simulink model "Final_Model_Building_2_AirflowAdded_BufferMode"  (R2022a)
settings: Solver=FixedStepAuto  StartTime=0.0  StopTime=24*3600  FixedStep=5  RelTol=1e-3
values from neighbouring files (symbols this model uses):
  Aux_Threshold = 52    [Setup_Code_EWASP_VC.m]
  buildingAge = 2005    [Setup_Code_EWASP_VC.m]
  ceilingHeight = 2.4    [Setup_Code_EWASP_VC.m]
  conductiveHconnectMatrix = [ ... (first row only)    [Setup_Code_EWASP_VC.m]
  cRoofGreen = 100000    [Setup_Code_EWASP_VC.m]
  Defrost_After_Time = 30    [Setup_Code_EWASP_VC.m]
  DHWDemandProfile = occFreegainHotwaterElecTestPassiveOcc3(:,3)    [Setup_Code_EWASP_VC.m]
  Elec_Max = Elec_Max*(30/24.2)    [Setup_Code_EWASP_VC.m]
  Elec_Mid = Elec_Mid*(30/24.2)    [Setup_Code_EWASP_VC.m]
  Elec_Min = Elec_Min*(30/24.2)    [Setup_Code_EWASP_VC.m]
  ElecDemandProfile = occFreegainHotwaterElecTestPassiveOcc3(:,4)    [Setup_Code_EWASP_VC.m]
  ElecFixed = [Elec_Max(6,2) Elec_Max(6,4) Elec_Max(6,6) Elec_Max(6,7) ... (first row only)    [Setup_Code_EWASP_VC.m]
  floorOrCeilingArea = floorOrCeilingArea*1.15    [Setup_Code_EWASP_VC.m]
  freegain = occFreegainHotwaterElecTestPassiveOcc3(:,2)-max(occupancy)*25    [Setup_Code_EWASP_VC.m]
  furnitureModelOn = 1    [Setup_Code_EWASP_VC.m]
  Heat_Max = Heat_Max*(30/24.2)    [Setup_Code_EWASP_VC.m]
  Heat_Mid = Heat_Mid*(30/24.2)    [Setup_Code_EWASP_VC.m]
  Heat_Min = Heat_Min*(30/24.2)    [Setup_Code_EWASP_VC.m]
  HeatFixed = [Heat_Max(6,2) Heat_Max(6,4) Heat_Max(6,6) Heat_Max(6,7) ... (first row only)    [Setup_Code_EWASP_VC.m]
  HeatingOnProfile = repmat(HeatingOnProfile,365,1)    [Setup_Code_EWASP_VC.m]
  HEX_ReturnLowerLimit = 52.5    [Setup_Code_EWASP_VC.m]
  HEX_ReturnUpperLimit = 55    [Setup_Code_EWASP_VC.m]
  LeakMultiplier = 1+(2*(rand()-0.5)/10)    [Setup_Code_EWASP_VC.m]
  maxOcc = max(occupancyProfile)    [Setup_Code_EWASP_VC.m]
  NESW_wallArea = max(NESW_Lengths*ceilingHeight-NESW_Windows,0)    [Setup_Code_EWASP_VC.m]
  NESW_Windows = [ ... (first row only)    [Setup_Code_EWASP_VC.m]
  numRooms = roomCount    [Setup_Code_EWASP_VC.m]
  occupancy = occupancyProfile    [Setup_Code_EWASP_VC.m]
  offsetDays = 0    [Setup_Code_EWASP_VC.m]
  overChargeSeries = repmat(overChargeSeries,365,1)    [Setup_Code_EWASP_VC.m]
  pumpChoice = pumpChoices(MinIndex,1)    [Setup_Code_EWASP_VC.m]
  pumpRamp = 180    [Setup_Code_EWASP_VC.m]
  RoofIrradiance = Flat_NS_EW_RoofIrradiance(:,1)    [Setup_Code_EWASP_VC.m]
  roofStartTemp = ones(11,1)*20    [Setup_Code_EWASP_VC.m]
  rooftype = 0    [Setup_Code_EWASP_VC.m]
  RoomDataMatrix = [zeros(1,12);ones(1,12)*wallDensity;zeros(1,12);ones(1,12)*wallU;ones(1,12)*windowU;ones(1,12)*floorU;ones(1,12)*ceilingU;zeros(1,12);windowArea, 0;floorOrCeilingArea;zeros(1,12);floorOrCeilingArea*ceilingHeight]    [Setup_Code_EWASP_VC.m]
  roomVol = roomVol*1.15    [Setup_Code_EWASP_VC.m]
  slabStartTemp = (GroundTempTimeSeries(offsetDays*1440+1,1)+thermostatSetting)/2    [Setup_Code_EWASP_VC.m]
  SlackRequest = zeros(1440,1)    [Setup_Code_EWASP_VC.m]
  SolarThermalExists = 0    [Setup_Code_EWASP_VC.m]
  SourceFixed = HeatFixed-ElecFixed    [Setup_Code_EWASP_VC.m]
  StateSeries = StateSeriesGenerator(22,7,1)    [Setup_Code_EWASP_VC.m]
  Tank_Lower_Temp = 49.5    [Setup_Code_EWASP_VC.m]
  Tank_Upper_Temp = 52    [Setup_Code_EWASP_VC.m]
  Tank_Volume_m3 = 0.15    [Setup_Code_EWASP_VC.m]
  TankHeatHour = randi([1 5])-1    [Setup_Code_EWASP_VC.m]
  upDown = [0;0;0;0;1;1;1;1;1;1;1]    [Setup_Code_EWASP_VC.m]
  wallStartTempExt = thermostatSetting*(0.266+0.00215*outdoorStartTemp+0.018*wallU+0.00113*outdoorStartTemp*wallU+0.0068*wallU^2)    [Setup_Code_EWASP_VC.m]
undefined symbols (not defined in the file or in its folder): a, ceilingU, condUDMatrix, convUDMatrix, deltaPEXPANDED_E, deltaPEXPANDED_E2, deltaPEXPANDED_N, deltaPEXPANDED_N2, deltaPEXPANDED_S, deltaPEXPANDED_S2, deltaPEXPANDED_W, deltaPEXPANDED_W2, DesiredDHWTemp, DesiredFlowTempVsInOutDeltaTemp, DiffuseHorizontal, DiscIntNeverNeededParam, DNI, dwnAndConcrete, ExtractRates, GroundTempTimeSeries, HCM, HCM2, HCM_closed, HCM_closed2, intermediateU, IsTop, massFlowMatrix, mechEfficiency, neighbourMatrix, numericalRoomUse, RadiatorMatrix, room2roomflowmatrix_E, room2roomflowmatrix_E2, room2roomflowmatrix_N, room2roomflowmatrix_N2, room2roomflowmatrix_S, room2roomflowmatrix_S2, room2roomflowmatrix_W, room2roomflowmatrix_W2, StateAirInEXPANDED_E, StateAirInEXPANDED_E2, StateAirInEXPANDED_N, StateAirInEXPANDED_N2, StateAirInEXPANDED_S, StateAirInEXPANDED_S2, StateAirInEXPANDED_W, StateAirInEXPANDED_W2, StateAirOutEXPANDED_E, StateAirOutEXPANDED_E2, StateAirOutEXPANDED_N, StateAirOutEXPANDED_N2, StateAirOutEXPANDED_S, StateAirOutEXPANDED_S2, StateAirOutEXPANDED_W, StateAirOutEXPANDED_W2, tankExists, TemperatureSeries, ThermostatBand, ThermostatSetting, Tin1 ... (+10)
libraries: simulink x6, dspsigops x4, dspmtrx3 x4, powerlib_meascontrol x3, carnot x3, dspstat3 x2
(part 7 of 29)

== system Final_Model_Building_2_AirflowAdded_BufferMode/GSHP_Subsystem/Subsystem3 ==
  note: only required to allow me to send the
      | same signal to 2 different outputs
  note: SH GSHP
  In1 : Inport
  In2 : Inport  Port=2
  In3 : Inport  Port=3
  In4 : Inport  Port=4
  In5 : Inport  Port=5
  In6 : Inport  Port=6
  In7 : Inport  Port=7
  Bus Selector1 : BusSelector  OutputSignals=Pelec  OutputAsBus=on
  Clock4 : Clock
  Data Type Conversion2 : DataTypeConversion  OutDataTypeStr=double  SaturateOnIntegerOverflow=off  RndMeth=Floor
  Data Type Conversion3 : DataTypeConversion  OutDataTypeStr=double  SaturateOnIntegerOverflow=off  RndMeth=Floor
  Data Type Conversion4 : DataTypeConversion  OutDataTypeStr=double  SaturateOnIntegerOverflow=off  RndMeth=Floor
  Ground_Source_Heat_Exchanger1 : Subsystem  AncestorBlock=carnot/Source/Heat_Pump/Ground_Source_Heat_Exchanger  mask(vertical ground source heat exchanger){Jahresmitteltemp_C=12, TGrad=0.025, lambdaErde=5, cpErde=11000, rhoErde=2500, lambdaFill=5, cpFill=1000, rhoFill=2000, Sondelaenge=100, B=10, Sondendurchmesser=0.032, Bohrdurchmesser=0.18, sondenfall=2 probes B/H = 0.1, np=2, DimAxi=10, DimRad=10, Gitterfaktor=2.5}
      mask prompts: Jahresmitteltemp_C "Average annual outdoor temperature  in °C"; TGrad "Temperature gradient in K/m, typical 0.025..0.04"; lambdaErde "Thermal conductivity ground in W/m/K"; cpErde "Heat capacity of the ground in J/kg/K"; rhoErde "Denstiy of the ground in kg/m³"; lambdaFill "Thermal conductivity filling in W/m/K"; cpFill "Heat capacity of the filling in J/kg/K"; rhoFill "Denstiy of the filling in kg/m³"; Sondelaenge "H: Length of earth probe in m"; B "B: probe distance in m"; Sondendurchmesser "Diameter of tube in m"; Bohrdurchmesser "Diameter of drilled hole in m"; sondenfall "Field geometry"; np "Number of parallel tubes"; DimAxi "No. of nodes in axial direction (typical 10)"; DimRad "No. of nodes in radial direction (typical 10)"; Gitterfaktor "grid factor (typical 2.5)"
      mask help:
      | The CARNOT EWS model is a transient model for dynamic simulation of borehole heat exchangers or so-called vertical ground heat exchangers. The model is based on the equations described by [Huber97] and has been implemented using the state space model of Matlab/Simulink [Bianchi06].
      | Bianchi M. A., Adaptive modellbasierte prädiktive Regelung einer Kleinwärmepumenanlage Diss. ETH Zuerich, No. 16892, 2006
      | Huber A, Schuler O., Berechnungsmodul für Erdwärmesonden (EWS). ENET Bericht Nr. 9658807-1, 1997
      mask init:
      | % Sets the parameters for the model
      | % ***********************************************************************
      | % This file is part of the CARNOT Blockset.
      | %   CARNOT is free software: you can redistribute it and/or modify
      | %   it under the terms of the GNU Lesser General Public License as published by
      | %   the Free Software Foundation, either version 3 of the License, or
      | %   (at your option) any later version.
      | %   CARNOT is distributed in the hope that it will be useful,
      | %   but WITHOUT ANY WARRANTY; without even the implied warranty of
      | %   MERCHANTABILITY or FITNESS FOR A PARTICULAR PURPOSE.  See the
      | %   GNU Lesser General Public License for more details.
      | %   You should have received a copy (copying_lesser.txt) of the 
      | %   GNU Lesser General Public License along with CARNOT.  
      | %   If not, see <http://www.gnu.org/licenses/>.
      | %  
      | % **********************************************************************
      | % author list:      fab -> Fabian Ochs
      | %                   hf  -> Bernd Hafner
      | %
      | % version: CarnotVersion.MajorVersionOfFunction.SubversionOfFunction
      | %
      | % Version  Author  Changes                                     Date
      | % 5.1.0    fab     created, based on Diss. Bianchi ETH Zurich  01dec2012
      | % 5.1.1    hf      adapted to carnot input and output struct.  04mar2013 
      | %
      | % Copyright (c) 2012 TU Insbruck, Fabian Ochs
      | 
      | startfall = 2; % 2: g-function
      | mdot = 0.5;
      | teta_in = 1;
      | Massenstrom = mdot/np;
      | Qdot0 = 5000;
      | t_start = 50*8560*3600;
      | 
      | % Geometry
      | Dicke_Sondenrohr = 0.003;
      | lambda_Sondenrohr = 0.48;
      | Bu = .1293;
      | 
      | % Ground Properties
      | aErde = lambdaErde/(rhoErde*cpErde);
      | 
      | % Fluid
      | teta_m = 2; 
      | p0 = 1E5;
      | fluid = 5;
      | mix = 0.25;
      | 
      | Jahresmitteltemp=Jahresmitteltemp_C + 273.15;
      | Bodenerwaermung=1;                          % 0°C
      | Bodentemp=Jahresmitteltemp+Bodenerwaermung; % K
      | 
      | % Calculation
      | lambdaSole=thermal_conductivity(teta_m,p0,fluid,mix);%W/(m K)
      | cpSole=heat_capacity(teta_m,p0,fluid,mix);                                % J/Kg*K
      | rhoSole=density(teta_m,p0,fluid,mix);%kg/m^3
      | vSole=kinematic_viscosity(teta_m,p0,fluid,mix);                             % m2/s
      | 
      | Pr=vSole*rhoSole*cpSole/lambdaSole;
      | rb = Bohrdurchmesser/2;
      | rm = B/2;
      | Rechenradius = rm;
      | Dl=Sondelaenge/DimAxi*2;    
      | 
      | rs=Sondendurchmesser/2;
      | r0 = rs-Dicke_Sondenrohr; % Innenradius
      | r1=Bohrdurchmesser/2;
      | r2=r1+(Rechenradius-r1)*(1-Gitterfaktor)/(1-Gitterfaktor^(DimRad-1))*Gitterfaktor^0;
      | 
      | rz1=((r1^2+r0^2)/2)^0.5;
      | rz2=((r2^2+r1^2)/2)^0.5;
      | 
      | mcpSole=2*cpSole*rhoSole*pi*Dl*(Sondendurchmesser/2)^2;
      | Di = Sondendurchmesser - 2 * Dicke_Sondenrohr;
      | Geschw_Sole= Massenstrom/rhoSole/(Di/2)^2/pi/2; % 2: double U
      | 
      | Vdot = Massenstrom/rhoSole;
      | A_p = (Di/2)^2/pi/2;
      | 
      | Re=Geschw_Sole*Di/vSole;
      | Druckverlust= 1/(1.82*log10(Re)-1.64)^2;
      | K1=1+27.2*Druckverlust/8;
      | K1_o=1.106886;
      | K2=11.7+1.8*Pr^(-1.3);
      | Druckverlust_o=0.031437;
      | St_o= Druckverlust_o/8/(K1_o+K2*(Druckverlust_o/8)^0.5*(Pr^(2/3)-1));
      | Nu_o=St_o*10000*Pr;
      | St= Druckverlust/8/(K1+K2*(Druckverlust/8)^0.5*(Pr^(2/3)-1));
      | 
      | % acc. Hellström    
      | b = Bu/(2*r1);
      | b_max = 1-rs/r1;
      | b_min = rs/r1;
      | sigma = (lambdaFill-lambdaErde)/(lambdaErde+lambdaFill);
      | A = pi*r0^2;
      | vs = Massenstrom/2/rhoSole/A;
      | zeta = 1/((1.82*log10(Re)-1.64)^2);
      | K1 = 1+27.2*zeta/8;
      | K2 = 11.7+1.8*Pr^(-1/3); 
      | R_s = 1/(2*pi*lambda_Sondenrohr)*log(rs/r0);
      |     
      | Nu_turbulent=St*Re*Pr;        
      | Nu_laminar=4.36;
      | 
      | if Re>=10000,
      |     Nu =(zeta/8)*Re*Pr/(K1+K2*(zeta/8)^.5*(Pr^(2/3)-1));
      | elseif Re<10000 && Re>2300
      |     Nu = Nu_laminar*exp(log(Nu_o/Nu_laminar)*log(Re/2300)/log(10000/2300));
      | elseif Re<=2300,
      |     Nu=Nu_laminar;        
      | end
      |     
      | alpha = Nu*lambdaSole/(2*r0);
      | alpha_eff = (1/alpha+r0/lambda_Sondenrohr*log(rs/r0))^-1;
      | alpha0 = lambdaSole/(Di/2*(1-0.5^0.5));
      | alpha0_eff = (1/alpha0+r0/lambda_Sondenrohr*log(rs/r0))^-1;
      | 
      | R_a = 1/(8*pi*alpha*r0);
      | beta = lambdaFill*(1/(r0*alpha)+1/lambda_Sondenrohr*log(rs/r0));
      | 
      | R1_EWS=0.25*(1/(2*pi*alpha_eff*r0*Dl)+1/(2*pi*lambdaFill*Dl)*log((r1-rz1)/r0));
      | R2_EWS=1/(2*pi*Dl)*(1/lambdaFill*log(r1/rz1)+1/lambdaErde*log(rz2/r1));        
      | R10_EWS=0.25*(1/(2*pi*alpha0_eff*r0*Dl)+1/(2*pi*lambdaFill*Dl)*log((r1-rz1)/r0));
      | R20_EWS=1/(2*pi*Dl)*(1/lambdaFill*log(r1/rz1)+1/lambdaErde*log(rz2/r1));        
      | 
      | Ra = 1/(pi*lambdaFill)*(log((2^.5*b*r1)/r0)-1/2*log((2*b*r1)/r0)-1/2*sigma*log((1-b^4)/(1+b^4)))+(1/(2*pi*r0*alpha))+R_s;
      | Rb = (1/(8*pi*lambdaFill))*(beta+log(r1/r0)+log(r1/Bu)+sigma*log(r1^4/(r1^4-Bu^4/16))-(r0^2/Bu^2*(1-sigma*(Bu^474)/(r1^4-Bu^4/16)^2))/((1+beta)/(1-beta)+r0^2/Bu^2*(1+sigma*Bu^4*r1^4/(r1^4-Bu^4/16)^2)));
      | Ra0 = 1/(pi*lambdaFill)*(log((2^.5*b*r1)/r0)-1/2*log((2*b*r1)/r0)-1/2*sigma*log((1-b^4)/(1+b^4)))+(1/(2*pi*r0*alpha0))+R_s;
      | Rb0 = (1/(8*pi*lambdaFill))*(beta+log(r1/r0)+log(r1/Bu)+sigma*log(r1^4/(r1^4-Bu^4/16))-(r0^2/Bu^2*(1-sigma*(Bu^474)/(r1^4-Bu^4/16)^2))/((1+beta)/(1-beta)+r0^2/Bu^2*(1+sigma*Bu^4*r1^4/(r1^4-Bu^4/16)^2)));
      | 
      | if Ra < 4 * Rb
      |     R1 = Ra/(4*Dl);
      |     R2 = (Rb-Ra/4)/Dl+(2*pi*Dl*lambdaErde)^-1*log(rz2/r1);
      |     R10 = Ra0/(4*Dl);
      |     R20 = (Rb0-Ra0/4)/Dl+(2*pi*Dl*lambdaErde)^-1*log(rz2/r1);        
      | else
      |     R1 = R1_EWS;
      |     R2 = R2_EWS;
      |     R10 = R10_EWS;
      |     R20 = R20_EWS;
      | end
      |     
      | % temperaturverlauf axialer richtung
      | L0=cpSole*Massenstrom;      % konstant
      | L00 = 0.0;
      | L1=1/R1;
      | L2=1/R2;
      | L10=1/R10;
      | L20=1/R20;
      | 
      | % matrizen Ad,Bd,Cd,Dd für Tdown
      | Ad=zeros(DimAxi/2,DimAxi/2);
      | Ad0=zeros(DimAxi/2,DimAxi/2);
      | for h=1:DimAxi/2,
      |     Ad(h,h)=-(L0/(mcpSole)+L1/(2*mcpSole));
      |     Ad0(h,h)=-(L00/(mcpSole)+L10/(2*mcpSole));
      | end
      |   
      | for h=1:DimAxi/2-1,
      |     Ad(h+1,h)=L0/(mcpSole);
      |     Ad0(h+1,h)=L00/(mcpSole);
      | end
      | 
      | Bd=zeros(DimAxi/2,DimAxi/2+1);
      | Bd0=zeros(DimAxi/2,DimAxi/2+1);
      | Bd(1,1)=L0/(mcpSole);
      | Bd0(1,1)=L00/(mcpSole);
      | 
      | for h=1:DimAxi/2,
      |     Bd(h,h+1)=L1/(2*mcpSole);
      |     Bd0(h,h+1)=L10/(2*mcpSole);
      | end
      | 
      | Cd=eye(DimAxi/2);
      | Dd=zeros(DimAxi/2,DimAxi/2+1);
      | 
      | % matrizen Au,Bu,Cu,Du für Tup
      | Au=zeros(DimAxi/2,DimAxi/2);
      | Au0=zeros(DimAxi/2,DimAxi/2);
      | for h=1:DimAxi/2,
      |     Au(h,h)=-(L0/(mcpSole)+L1/(2*mcpSole));
      |     Au0(h,h)=-(L00/(mcpSole)+L10/(2*mcpSole));
      | end
      |   
      | for h=1:DimAxi/2-1,
      |     Au(h+1,h)=L0/(mcpSole);
      |     Au0(h+1,h)=L00/(mcpSole);
      | end
      | 
      | Bu=zeros(DimAxi/2,DimAxi/2+1);
      | Bu0=zeros(DimAxi/2,DimAxi/2+1);
      | Bu(1,1)=L0/(mcpSole);
      | Bu0(1,1)=L00/(mcpSole);
      | for h=1:DimAxi/2,
      |     Bu(h,h+1)=L1/(2*mcpSole);
      |     Bu0(h,h+1)=L10/(2*mcpSole);
      | end
      | 
      | Cu=Cd;
      | Du=zeros(DimAxi/2,DimAxi/2+1);
      | 
      | % berechnung von Tradial, von Luzi Valär
      | Dim1=(DimRad-2)*DimAxi/2;
      | r = zeros(1:DimRad);
      | r(1)=Bohrdurchmesser/2;
      | r(2)=r2;
      | for h =3:DimRad,
      |     r(h)=r(h-1)+(Rechenradius-r1)*(1-Gitterfaktor)/(1-Gitterfaktor^(DimRad-1))*Gitterfaktor^(h-2);
      | end
      |     
      | rz = zeros(1:DimRad);
      | rz(1)=((r(1)^2+r0^2)/2)^0.5;
      | for h = 2:DimRad,
      |     rz(h)=((r(h)^2+r(h-1)^2)/2)^0.5;
      | end
      | 
      | L = zeros(1:DimRad);
      | L(1)=L1; 
      | L(2)=L2;
      | for h = 3:DimRad-1,
      |     L(h)=1/(1/(2*pi*Dl)*(1/lambdaErde*log(rz(h)/rz(h-1))));
      | end
      | L(DimRad)=1/(1/(2*pi*Dl)*(1/lambdaErde*log(r(DimRad)/rz(DimRad-1))));
      | 
      | 
      | C = zeros(1:DimRad);
      | C(1)=cpFill*rhoFill*pi*(r(1)^2-4*r0^2)*Dl;
      | for h = 2:DimRad,
      |     C(h)=cpErde*rhoErde*pi*(r(h)^2-r(h-1)^2)*Dl;
      | end
      | 
      | 
      | a=zeros(DimRad-2,DimRad-2);
      | for h = 1:DimRad-2,
      |     a(h,h)=(-L(h)-L(h+1))/C(h);
      | end
      | for h = 1:DimRad-3,
      |     a(h,h+1)=L(h+1)/C(h);
      |     a(h+1,h)=L(h+1)/C(h+1);
      | end
      | 
      | b=zeros(DimRad-2,2);
      |     b(1,1)=L(1)/C(1);
      |     b(DimRad-2,2)=L(DimRad-1)/C(DimRad-2);
      |     
      | %%%%%%%%%%%%%%%%%%%%%%%%%%%%%%%%%%%%%%%%%%%%%%%%%%% 
      |     
      | Ar=a;
      | Ar(DimRad-1:2*(DimRad-2),DimRad-1:2*(DimRad-2))=a;
      |     
      | for h=2:DimAxi/2-1,
      |     Ar(h*(DimRad-2)+1:(h+1)*(DimRad-2),h*(DimRad-2)+1:(h+1)*(DimRad-2))=a;
      | 
      | end  
      | 
      | Br=b;
      | 
      | for h=1:DimAxi/2-1,
      |     Br(h*(DimRad-2)+1:(h+1)*(DimRad-2),2*h+1:2*h+2)=b;   
      | end
      |     
      | 
      | Cr=eye((DimRad-2)*DimAxi/2);
      | Dr=zeros((DimRad-2)*DimAxi/2,DimAxi);
      | 
      | % andere matrizen
      | Cdl=zeros(DimAxi/2,1);
      | Cdl(DimAxi/2,1)=1;
      | Cdl=Cdl';
      | 
      | c1=zeros(DimAxi/2,Dim1);
      | for h=1:DimAxi/2,
      |     c1(1,1)=1;
      |     c1(h,(h-1)*(DimRad-2)+1)=1;
      | end
      | 
      | c31=zeros(1,DimAxi/2);
      | c3(1,1)=1;
      | for h=1:DimAxi/2-1,
      |     c3(1+2*h,1+h)=1;
      | end
      | 
      | c33=zeros(DimAxi,DimAxi/2);
      | c33(1:DimAxi-1,1:DimAxi/2)=c3;
      | 
      | c41=zeros(1,DimAxi/2);
      | c4=c41;
      | c4(2:DimAxi,1:DimAxi/2)=c3;
      | 
      | 
      | % randbedingungen für Tearth,DimRad
      | % anfangsbedingungen für Tradial
      | mu=linspace(0,Sondelaenge,DimAxi/2);
      | T=(mu*TGrad+Bodentemp);
      | Tearth_anf=T'*ones(1,DimRad-2);
      | T_null=Tearth_anf(:,1);
      | teta_fluid_ini = mean(T_null)-273.15;
      | 
      | % anfangsbedingungen für Tdown,Tup
      | Tdown_0=Tearth_anf(:,1);
      | Tup_0=flipud(Tdown_0);
      | Tearth_anf=Tearth_anf';
      | c5=ones(DimAxi/2,1);           
      | 
      | c6=zeros(DimRad-2,3*(DimRad-2));
      | 
      | for i=2:DimRad-2;
      |     c6(1,DimRad-1)=1;
      |     c6(i,DimRad+i-2)=1;
      | end
      | 
      | %% RB
      | Ts_Trichter=7*24*3600; % 7 (1 week according to Huber)
      | Dr_Trichter=1;
      | t_Trichter = linspace(Ts_Trichter,Ts_Trichter*5000,5000);
      | r_Trichter = linspace(Dr_Trichter,Dr_Trichter*20,20);
      | 
      | % g-function
      | xS = [-4 -2 0 2 3];
      | if sondenfall == 1          % 1 Sonde
      |     yS = [4.82 5.69 6.29 6.57 6.6];
      | elseif sondenfall == 2      % 2 Sonden B/H = 0.1
      |     yS = [4.99 6.37 7.62 8.06 8.08];
      | elseif sondenfall == 3      % 2 Sonden B/H = 0.05
      |     yS = [5.30 6.92 8.20 8.67 8.71];
      | elseif sondenfall == 4      % 3x6 Sonden B/H = 0.1
      |     yS = [5.00 9.15 16.40 19.75 20.05];
      | elseif sondenfall == 5      % 5x10 Sonden B/H = 0.1
      |     yS = [5.00 10.2 22.75 29.5 30.05];
      | end
      | 
      | npol = 4;
      | p = polyfit(xS,yS,npol);
      | ts = Sondelaenge^2/(9*aErde);
      | gfunction = zeros(length(t_Trichter),length(r_Trichter));
      | Es = t_Trichter*9*aErde/Sondelaenge^2;
      | 
      | g = polyval(p,log(Es));
      | 
      | for ii = 1:length(r_Trichter)
      |     gfunction(:,ii) = max(0,g - log(r_Trichter(ii)/Sondelaenge/0.0005)); % correction 21-09-2012
      | end
      | 
      | % Startwerte
      | qdot0 = Qdot0/Sondelaenge; 
      | if startfall == 2
      |     Es_start = t_start*9*aErde/Sondelaenge^2;
      |     TEarth0 = zeros(size(Tearth_anf));
      |     for ii = 1:DimAxi/2
      |         for iii = 1:DimRad-1
      |             g_start = polyval(p,log(Es_start));
      |             TEarth0(iii,ii) = Bodentemp + mu(ii)*TGrad - qdot0/(DimAxi/2)*((g_start-log(rz(iii+1)/Sondelaenge/0.0005))/(2*pi*lambdaErde));
      |         end
      |     end    
      | 
      |     T_null = TEarth0(end,:)';
      |     Tearth_anf = TEarth0(1:end-1,:);
      | end
      mask Help: web(['file:///' fullfile(path_carnot('help'),'Ground_Source_Heat_Exchanger.html')],'-helpbrowser')
      mask TypeOptions sondenfall: 1 probe | 2 probes B/H = 0.1 | 2 probes B/H = 0.05 | 3x6 probes B/H = 0.1 | 5x10 probes B/H = 0.1
      mask DialogControl ParameterTabVar0 Prompt: General
      mask DialogControl ParameterTabVar01 Prompt: Geometry
      mask DialogControl ParameterTabVar012 Prompt: Calculation
      mask Display:
      | plot(0,10,100,90,[70,30],[80,80],[35,35,43,43,47,52,57,57,66,66,60,60,54,46,40,40,35],[84,87,87,20,13,13,21,87,87,84,84,20,10,10,20,84,84])
      | port_label('input',1,'Tin')
      | port_label('input',2,'Mdot')
      | port_label('output',1,'THB')
      | port_label('output',2,'Tn')
  HeatPump_Simplified : Subsystem  AncestorBlock=carnot/Source/Heat_Pump/HeatPump  mask(heat pump){Tcin=[-5 7 12], Thout=[35 45 55 60], Qdotc=[4400*a-2000*a 4200*a-2000*a 3200*a-2000*a 1800*a-2000*a;5800*a-2100*a 5500*a-2100*a 4200*a-2100*a 2800*a-2100*a;8400*a-2200*a 7200*a-2200*a 5500*a-2200*a 3300*a-2200*a], Qdoth=[4400*a 4200*a 3200*a 1800*a;5600*a 5500*a 4200*a 2800*a;8400*a 7200*a 5500*a 3300*a], Pel=[2000*a 2000*a 2000*a 2000*a;2100*a 2100*a 2100*a 2100*a;2200*a 2200*a 2200*a 2200*a], caph=10*4180, capc=4180*225, UA=2, linc=10, quac=10, linh=10, quah=10}
      mask prompts: Tcin "inlet source temperature vector (°C)"; Thout "outlet load temperature vector (°C)"; Qdotc "source power matrix (W)"; Qdoth "heating power matrix (W)"; Pel "electric power matrix (W)"; caph "thermal capacity hot loop [J/K]"; capc "thermal capacity cold loop [J/K]"; UA "heat loss coefficient [W/K]"; linc "Cold side linear massflow dependant pressure drop in [Pa*s/kg]"; quac "Cold side quadratic massflow dependant pressure drop hot side in [Pa*s²/kg]"; linh "Hot side linear massflow dependant pressure drop in [Pa*s/kg]"; quah "Hot side quadratic massflow dependant pressure drop hot side in [Pa*s²/kg]"
      mask help:
      | Linearized heat pump model. Uses measured data according to EN 14511 as input.
      | heating power: Qdot_h = K1*Tcold_in + K2*Thot_out + K3
      | electric power: Pel = K4*Tcold_in + K5*Thot_out + K6
      | source power: Qdot_c = -K7*Tcold_in - K8*Thot_out - K9
      | differential equation: cap*dTh/dt = Qdot + mdot*cp*(T_in-T) + UA*(Tamb-T)
      | with: cap = mass * heat_capactiy
      | See hp_param.m for the parameters K1 to K9.
      | Literature: Schwamberger, K.: Fortschrittsberichete VDI, Nr. 263, 1991
      mask init: same as Final_Model_Building_2_AirflowAdded_BufferMode/ASHP_Subsystem/DHW for ASHP Case/HeatPump_Simplified1
      mask Help: web(fullfile(path_carnot('help'),'heatpump.html'),'-helpbrowser')
      mask DialogControl ParameterTabVar0 Prompt: HP Caracteristic
      mask DialogControl ParameterTabVar01 Prompt: Thermal
      mask DialogControl ParameterTabVar012 Prompt: Hydraulic
      mask Display: plot(-20,-10,120,110,[10,20,40,60,80,90,90,80,60,40,20,10,10],[60,80,90,90,80,60,40,20,10,10,20,40,60],[40,20],[90,20],[60,80],[90,20],[50,50],[30,50],[60,40],[40,40],[57,43],[33,46],[44,57],[34,46])
  Instantaneous to kWh Total2 : Subsystem
  Logical Operator : Logic  Operator=NOT  AllPortsSameDT=off  OutDataTypeStr=boolean
  Logical Operator1 : Logic  AllPortsSameDT=off  OutDataTypeStr=boolean
  Logical Operator2 : Logic  Operator=NOT  AllPortsSameDT=off  OutDataTypeStr=boolean
  Logical Operator3 : Logic  Operator=OR  AllPortsSameDT=off  OutDataTypeStr=boolean
  Logical Operator6 : Logic  AllPortsSameDT=off  OutDataTypeStr=boolean
  Massflow when system is off : Constant  Value=0
  Massflow when system is off1 : Constant  Value=0
  Massflow when system is on : Constant  Value=3400/3600
  Plus : Sum
  Scope3 : Scope
  Switch1 : Switch  Criteria=u2 > Threshold  Threshold=0.5  SaturateOnIntegerOverflow=off  InputSameDT=off
  Switch5 : Switch  Criteria=u2 > Threshold  Threshold=0.5  SaturateOnIntegerOverflow=off  InputSameDT=off
  Switch6 : Switch  Criteria=u2 > Threshold  Threshold=10  SaturateOnIntegerOverflow=off  InputSameDT=off
  Terminator8 : Terminator
  on? (I/O)9 : Constant  Value=20  OutDataTypeStr=double
  tank_sensor_temp4 : Scope
  tank_sensor_temp5 : Scope
  x : Constant  Value=0
  Out1 : Outport  VectorParamsAs1DForOutWhenUnconnected=off
  Out2 : Outport  Port=2  VectorParamsAs1DForOutWhenUnconnected=off
  Out3 : Outport  Port=3  VectorParamsAs1DForOutWhenUnconnected=off
  Out4 : Outport  Port=4  VectorParamsAs1DForOutWhenUnconnected=off
  Out5 : Outport  Port=5  VectorParamsAs1DForOutWhenUnconnected=off
  Out6 : Outport  Port=6  VectorParamsAs1DForOutWhenUnconnected=off
  Out7 : Outport  Port=7  VectorParamsAs1DForOutWhenUnconnected=off
  Out8 : Outport  Port=8  VectorParamsAs1DForOutWhenUnconnected=off
  tag scope: HeatPumpFlow=global
  wires:
  In2/1 -> [MixedTemp]
  [pump_power_Fraction] -> HeatPump_Simplified/7(power fraction)
  Switch6/1 -> HeatPump_Simplified/2(THB_r)
  Logical Operator/1 -> Logical Operator6/2
  x/1 -> Plus/2
  Massflow when system is on/1 -> Switch1/1
  Ground_Source_Heat_Exchanger1/2(Tnodes) -> tank_sensor_temp4/1, Terminator8/1
  HeatPump_Simplified/4(Real P_Therm) -> Out4/1, Instantaneous to kWh Total2/1(In1)
  Ground_Source_Heat_Exchanger1/1(Tout) -> Out8/1, [FromGround]
  [T_Out] -> HeatPump_Simplified/3(Tamb)
  [Global_Control_Signal] -> Logical Operator1/1
  Data Type Conversion2/1 -> Out1/1, Plus/1, HeatPump_Simplified/4(Ctrl)
  HeatPump_Simplified/1(T_source) -> Out6/1
  Bus Selector1/1 -> Out5/1
  In3/1 -> [MassFlowTotal]
  Clock4/1 -> Switch6/2
  Switch5/1 -> HeatPump_Simplified/6(mdot_hot), [HeatPumpFlow], Out7/1, tank_sensor_temp5/1
  on? (I/O)9/1 -> Switch6/3
  HeatPump_Simplified/2("T_out ") -> Out3/1
  [DHW_on] -> Logical Operator3/2
  [Global_Control_Signal] -> Logical Operator6/1
  [Global_Control_Signal] -> Logical Operator3/1
  Switch1/1 -> [mdot_cold], Ground_Source_Heat_Exchanger1/2(Mdotin1)
  In1/1 -> [T_Out]
  Logical Operator3/1 -> Data Type Conversion4/1
  Massflow when system is off1/1 -> Switch5/3
  HeatPump_Simplified/3(HPdat) -> Bus Selector1/1
  [ToGroundTot] -> Ground_Source_Heat_Exchanger1/1(Tin)
  In4/1 -> [Global_Control_Signal]
  Data Type Conversion4/1 -> Switch1/2
  Logical Operator2/1 -> Logical Operator1/2
  [DHW_on] -> Logical Operator/1
  [MixedTemp] -> Switch6/1
  Massflow when system is off/1 -> Switch1/3
  Logical Operator6/1 -> Data Type Conversion2/1
  [MassFlowTotal] -> Switch5/1
  [mdot_cold] -> HeatPump_Simplified/5(mdot_cold)
  Instantaneous to kWh Total2/1(Out1) -> Scope3/1
  Logical Operator1/1 -> Data Type Conversion3/1
  In5/1 -> [pump_power_Fraction]
  [FromGround] -> HeatPump_Simplified/1(THBsource)
  Data Type Conversion3/1 -> Switch5/2
  In6/1 -> Logical Operator2/1
  In7/1 -> [ToGroundTot]
  Plus/1 -> Out2/1

== system Final_Model_Building_2_AirflowAdded_BufferMode/Subsystem3/Select correct element from array, considering offset6 ==
  In1 : Inport
  Clock1 : Clock
  Direct Lookup Table (n-D)1 : LookupNDDirect  NumberOfTableDimensions=1  TableIsInput=on
  Divide1 : Product  Inputs=*/
  Floor : Rounding
  Saturation2 : Saturate  UpperLimit=inf  LowerLimit=0
  Scope23 : Scope
  Sum : Sum  Inputs=|++
  on? (I/O)1 : Constant  Value=offsetDays*3600*24  OutDataTypeStr=double
  on? (I/O)3 : Constant  Value=60  OutDataTypeStr=double
  Out1 : Outport  VectorParamsAs1DForOutWhenUnconnected=off
  wires:
  Saturation2/1 -> Scope23/1, Direct Lookup Table (n-D)1/1
  on? (I/O)3/1 -> Divide1/2
  Divide1/1 -> Floor/1
  Floor/1 -> Saturation2/1
  Clock1/1 -> Sum/1
  Direct Lookup Table (n-D)1/1 -> Out1/1
  In1/1 -> Direct Lookup Table (n-D)1/2
  on? (I/O)1/1 -> Sum/2
  Sum/1 -> Divide1/1

== system Final_Model_Building_2_AirflowAdded_BufferMode/Subsystem4/Heatloss roof to environment ==
  In1 : Inport
  In2 : Inport  Port=2
  In3 : Inport  Port=3
  Subtract6 : Sum  Inputs=2
  Subtract7 : Sum  Inputs=+-
  Total roofstructure heat capacity1 : Product
  Total roofstructure heat capacity2 : Product  Inputs=3
  constants : Constant  Value=3
  constants1 : Constant  Value=2.8
  roofArea : Constant  Value=sum(floorOrCeilingArea(1,1:11)'.*IsTop(1,1:11)')*1.414
  Out1 : Outport  VectorParamsAs1DForOutWhenUnconnected=off
  wires:
  In3/1 -> Subtract7/1
  constants1/1 -> Subtract6/2
  Subtract6/1 -> Total roofstructure heat capacity2/1
  In2/1 -> Subtract7/2
  roofArea/1 -> Total roofstructure heat capacity2/3
  Total roofstructure heat capacity1/1 -> Subtract6/1
  constants/1 -> Total roofstructure heat capacity1/2
  Subtract7/1 -> Total roofstructure heat capacity2/2
  In1/1 -> Total roofstructure heat capacity1/1
  Total roofstructure heat capacity2/1 -> Out1/1

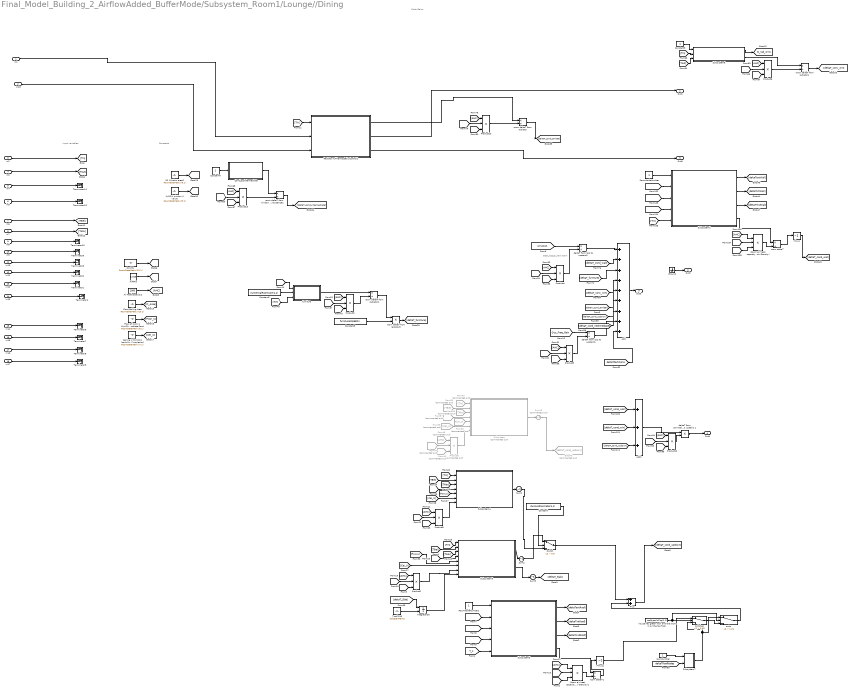
== system Final_Model_Building_2_AirflowAdded_BufferMode/Subsystem_Room1/Lounge//Dining ==
  note: Input variables
  note: Solar Gains
  note: Qdot_lost_to_next room
  note: Constants
  In1 : Inport
  In18 : Inport  Port=2
  In2 : Inport  Port=3
  In3 : Inport  Port=4
  In4 : Inport  Port=5
  In5 : Inport  Port=6
  In6 : Inport  Port=7
  In7 : Inport  Port=8
  In8 : Inport  Port=9
  In9 : Inport  Port=10
  In10 : Inport  Port=11
  In11 : Inport  Port=12
  In12 : Inport  Port=13
  In13 : Inport  Port=14
  In14 : Inport  Port=15
  In15 : Inport  Port=16
  In16 : Inport  Port=17
  In17 : Inport  Port=18
  Add : Sum  Inputs=+++++++++
  Add1 : Sum  Inputs=+++
  Air heat capacity2 : Constant  Value=1000
  AirRHO : Constant  Value=1.025
  "Ceiling U W/m2/k1 (could be intermediate floor, roof insulation)" : Constant  Value=RoomDataMatrix(7,1)
  CondLossIntermediate : Subsystem
      mask Display:
      | port_label('input',1, 'RoomNum')
      | port_label('output',1,'IntCondGain')
  Constant : Constant  Value=dwnAndConcrete(1,1)
  Constant2 : Constant  Value=numericalRoomUse(1,1)
  Constant3 : Constant
  Constant4 : Constant
  Constant5 : Constant  Value=furnitureModelOn
  Floor of room U W/m2/k (could be ground or intermediate floor) : Constant  Value=RoomDataMatrix(6,1)
  Floor/Ceiling Area : Constant  Value=RoomDataMatrix(10,1)
  From45 : From  Commented=on  GotoTag=Tin
  From46 : From  Commented=on  GotoTag=AHC
  From47 : From  Commented=on  GotoTag=RmVol
  From48 : From  Commented=on  GotoTag=AirRHO
  From55 : From  Commented=on  GotoTag=TBel
  From56 : From  Commented=on  GotoTag=TAbv
  From57 : From  Commented=on  GotoTag=Fl_Area
  From58 : From  Commented=on  GotoTag=Floor_U
  From59 : From  Commented=on  GotoTag=Cei_U
  Goto43 : Goto  Commented=on  GotoTag=deltaT_cond_updown
  Ground : Ground
  Integrator26 : Integrator  InitialConditionSource=external  InitialCondition=Tin1
  M2 Window area2 : Constant  Value=RoomDataMatrix(9,1)
  Minus : Sum  Inputs=-
  Minus1 : Sum  Inputs=-
  Plus : Sum
  Product{1..6,10,12..13} (9 alike) : Product  Inputs=***
  Product8 : Product  Commented=on  Inputs=***
  Radiator w/Thermostatic Control2 : Subsystem  mask{DeltaT_Nominal=RadiatorMatrix(1,1), Power_Nominal=RadiatorMatrix(2,1), TRV_Therm_Setpoint=RadiatorMatrix(3,1), Water_Volume=RadiatorMatrix(4,1)}
      mask prompts: DeltaT_Nominal "DeltaT_Nominal (oC)"; Power_Nominal "Power_Nominal (W)"; TRV_Therm_Setpoint "TRV/Thermostat Setpoint (oC)"; Water_Volume "Water Volume (l)"
      mask Display:
      | disp('Radiator')
      | port_label('input', 1, 'Troom')
      | port_label('input', 2, 'Water Temp In')
      | port_label('input', 3, 'Water Mass Flow Rate (open)')
      | port_label('output', 1, 'Qdot2room')
      | port_label('output', 2, 'Water Temp Out')
      | port_label('output', 3, 'Actual Mass Flow')
      | %image('C:\Users\cpp14rcj\Desktop\MODEL IMAGES\radiator-67-778961.png')
  RmVOL : Constant  Value=RoomDataMatrix(12,1)
  Room air heat capacity (Cp*volume air*air Density) : Product  Inputs=***
  Room air heat capacity (Cp*volume air*air Density)1 : Product  Inputs=***
  RoomNodeNumber : Constant
  RoomNodeNumber1 : Constant
  Subsystem : Subsystem  Commented=on
      mask Display:
      | port_label('input',1,'T_in')
      | port_label('input',2,'T_below')
      | port_label('input',3,'T_above')
      | port_label('input',4,'Floor/Ceil Area')
      | port_label('input',5,'Floor U Value')
      | port_label('input',6,'Ceil U Value')
      | port_label('input',7,'Room Heat Capacity')
      | port_label('output',1,'deltaT_BF_cond')
      | disp('CBF')
  Subsystem1 : Subsystem  TreatAsAtomicUnit=on  SystemSampleTime=10
      mask Display:
      | disp('Wall Node \n Sub-Model')
      | port_label('input', 1, 'Room Node #')
      | port_label('input', 2, 'dT Internal NEWS in')
      | port_label('input', 3, 'dT Mid NEWS in')
      | port_label('input', 4, 'dT External NEWS in')
      | port_label('input', 5, 'T_Room')
      | port_label('output', 1, 'dT Internal NEWS out')
      | port_label('output', 2, 'dT Mid NEWS out')
      | port_label('output', 3, 'dT External NEWS out')
      | port_label('output', 4, 'Total Qloss Through Walls')
  Subsystem3 : Subsystem  SystemSampleTime=10
      mask Display:
      | disp('Roof Node \n Sub-Model')
      | port_label('input', 1, 'Room Node #')
      | port_label('input', 2, 'dT Internal NEWS in')
      | port_label('input', 3, 'dT Mid NEWS in')
      | port_label('input', 4, 'dT External NEWS in')
      | port_label('input', 5, 'T_Room')
      | port_label('output', 1, 'dT Internal NEWS out')
      | port_label('output', 2, 'dT Mid NEWS out')
      | port_label('output', 3, 'dT External NEWS out')
      | port_label('output', 4, 'Total Qloss Through Walls')
  Subsystem4 : Subsystem
      mask Display:
      | port_label('input',1,'T_in')
      | port_label('input',2,'T_below')
      | port_label('input',3,'T_above')
      | port_label('input',4,'Floor/Ceil Area')
      | port_label('input',5,'Floor U Value')
      | port_label('input',6,'Ceil U Value')
      | port_label('input',7,'Room Heat Capacity')
      | port_label('output',1,'deltaT_BF_cond')
      | disp('CBF')
  Subsystem5 : Subsystem
      mask Display:
      | port_label('input',1,'T_in')
      | port_label('input',2,'T_below')
      | port_label('input',3,'T_above')
      | port_label('input',4,'Floor/Ceil Area')
      | port_label('input',5,'Slab U Value')
      | port_label('input',6,'Ceil U Value')
      | port_label('input',7,'Room Heat Capacity')
      | port_label('input',8,'Slab Temp')
      | port_label('output',1,'deltaT_BF_cond')
      | port_label('output',2,'deltaT_Concrete')
      | disp('CBF_Concrete')
  Subsystem6 : Subsystem
      mask Display:
      | disp('Window Node \n Sub-Model')
      | port_label('input', 1, 'Room Node #')
      | port_label('input', 2, 'T_in')
      | port_label('input', 3, 'T_out')
      | port_label('output', 1, 'Qdot_winRad')
  Subsystem7 : Subsystem
  Sum1 : Sum  Inputs=-
  Sum13 : Sum  Commented=on  Inputs=-
  Sum2 : Sum  Inputs=-
  Sum5 : Sum  Inputs=-
  Switch : Switch  Criteria=u2 > Threshold  Threshold=0.5  SaturateOnIntegerOverflow=off  InputSameDT=off
  Terminator{1..12} (12 alike) : Terminator
  Twall136 : Constant  Value=slabStartTemp
  W/M2/k window U value : Constant  Value=RoomDataMatrix(5,1)
  deltaT from convective loss to upstairs 1 : Product  Inputs=**
  deltaT from loss to upstairs1 : Product  Inputs=*/
  deltaT from loss to upstairs2 : Product  Inputs=*/
  furniture : Subsystem
  "house has green roof, and the room is on the top floor" : Constant  Value=rooftype*IsTop(1,1)
  room deltaT : Product  Inputs=*/
  room deltaT from radiator : Product  Inputs=*/
  room deltaT from radiator1 : Product  Inputs=*/
  room deltaT from radiator2 : Product  Inputs=*/
  room deltaT from radiator3 : Product  Inputs=**
  room deltaT from window conductance1 : Product  Inputs=*/
  room deltaT1 : Product  Inputs=*/
  roomNumber : Constant
  switc : Switch  Criteria=u2 > Threshold  Threshold=1.01  SaturateOnIntegerOverflow=off  InputSameDT=off
  "switches " : Switch  Criteria=u2 > Threshold  Threshold=0.99  SaturateOnIntegerOverflow=off  InputSameDT=off
  Out1 : Outport  VectorParamsAs1DForOutWhenUnconnected=off
  Out2 : Outport  Port=2  VectorParamsAs1DForOutWhenUnconnected=off
  Out3 : Outport  Port=3  VectorParamsAs1DForOutWhenUnconnected=off
  Out4 : Outport  Port=4  VectorParamsAs1DForOutWhenUnconnected=off
  Out5 : Outport  Port=5  VectorParamsAs1DForOutWhenUnconnected=off
  tag scope: Q_rad_win1=global
  wires:
  In11/1 -> Terminator2/1
  In14/1 -> Terminator6/1
  From57/1 -> Subsystem/4(In4)
  [AirRHO] -> Product4/3
  Product8/1 -> Subsystem/7(In7)
  Add/1 -> Out3/1
  In15/1 -> Terminator7/1
  In8/1 -> Terminator10/1
  [deltaT_cond_updown] -> Add/6
  In5/1 -> Terminator12/1
  From48/1 -> Product8/3
  Sum13/1 -> Goto43/1
  In12/1 -> Terminator1/1
  deltaT from loss to upstairs2/1 -> Add/1
  In16/1 -> Terminator8/1
  In17/1 -> Terminator9/1
  From47/1 -> Product8/2
  From59/1 -> Subsystem/6(In6)
  Product4/1 -> deltaT from loss to upstairs2/2
  In3/1 -> [Tout]
  [AHC] -> Product4/1
  [AirLoss1] -> deltaT from loss to upstairs2/1
  From58/1 -> Subsystem/5(In5)
  [deltaT_cond_wall] -> Add/2
  In4/1 -> Terminator11/1
  From56/1 -> Subsystem/3(In3)
  Subsystem/1(Out1) -> Sum13/1
  In7/1 -> [TAbv]
  [RmVol] -> Product4/2
  In2/1 -> [Tin]
  From46/1 -> Product8/1
  From55/1 -> Subsystem/2(In2)
  From45/1 -> Subsystem/1(In1)
  [deltaT_conv_win] -> Add/4
  In9/1 -> Terminator5/1
  In6/1 -> [TBel]
  In10/1 -> Terminator3/1
  [RmVol] -> Product12/2
  [AirRHO] -> Product12/3
  [AHC] -> Product12/1
  deltaT from convective loss to upstairs 1/1 -> Out4/1
  [deltaT_cond_wall] -> Add1/1
  [deltaT_cond_win] -> Add1/2
  [deltaT_cond_updown] -> Add1/3
  Add1/1 -> deltaT from convective loss to upstairs 1/1
  Product12/1 -> deltaT from convective loss to upstairs 1/2
  [deltaT_cond_emitter] -> Add/5
  [RmVol] -> Product10/2
  room deltaT from radiator/1 -> [deltaT_cond_emitter]
  Radiator w/Thermostatic Control2/1(Out3) -> room deltaT from radiator/1
  Radiator w/Thermostatic Control2/2(Out1) -> Out1/1
  [AirRHO] -> Product10/3
  Product10/1 -> room deltaT from radiator/2
  [AHC] -> Product10/1
  In18/1 -> Radiator w/Thermostatic Control2/3(In2)
  [Tin] -> Radiator w/Thermostatic Control2/1(In1)
  In1/1 -> Radiator w/Thermostatic Control2/2(In3)
  Radiator w/Thermostatic Control2/3(Out2) -> Out5/1
  "Ceiling U W/m2/k1 (could be intermediate floor, roof insulation)"/1 -> [Cei_U]
  AirRHO/1 -> [AirRHO]
  Floor of room U W/m2/k (could be ground or intermediate floor)/1 -> [Floor_U]
  Air heat capacity2/1 -> [AHC]
  RmVOL/1 -> [RmVol]
  W/M2/k window U value/1 -> [Win_U]
  Floor/Ceiling Area/1 -> [Fl_Area]
  M2 Window area2/1 -> [win_Area]
  CondLossIntermediate/1(Out1) -> room deltaT from window conductance1/1
  Constant4/1 -> CondLossIntermediate/1(In1)
  [AirRHO] -> Product13/3
  [AHC] -> Product13/1
  Product13/1 -> room deltaT from window conductance1/2
  [RmVol] -> Product13/2
  room deltaT from window conductance1/1 -> [deltaT_cond_intermediate]
  [deltaT_cond_intermediate] -> Add/7
  RoomNodeNumber/1 -> Subsystem1/1(In1)
  Subsystem1/4(Out4) -> room deltaT/1
  [deltaTextWall] -> Subsystem1/4(In4)
  Subsystem1/1(Out1) -> [deltaTextWall]
  [deltaTmidWall] -> Subsystem1/3(In3)
  [deltaTintWall] -> Subsystem1/2(In2)
  Subsystem1/3(Out3) -> [deltaTmidWall]
  Subsystem1/2(Out2) -> [deltaTintWall]
  [Tin] -> Subsystem1/5(In5)
  [AirRHO] -> Room air heat capacity (Cp*volume air*air Density)/3
  [RmVol] -> Room air heat capacity (Cp*volume air*air Density)/2
  [AHC] -> Room air heat capacity (Cp*volume air*air Density)/1
  Room air heat capacity (Cp*volume air*air Density)/1 -> room deltaT/2
  room deltaT/1 -> Minus/1
  Minus/1 -> [deltaT_cond_wall]
  In13/1 -> Terminator4/1
  Ground/1 -> Out2/1
  Subsystem3/1(Out1) -> [deltaTextRoof]
  [deltaTintRoof] -> Subsystem3/2(In2)
  [AirRHO] -> Room air heat capacity (Cp*volume air*air Density)1/3
  Room air heat capacity (Cp*volume air*air Density)1/1 -> room deltaT1/2
  Subsystem3/2(Out2) -> [deltaTintRoof]
  room deltaT1/1 -> Minus1/1
  Subsystem3/3(Out3) -> [deltaTmidRoof]
  [deltaTmidRoof] -> Subsystem3/3(In3)
  [RmVol] -> Room air heat capacity (Cp*volume air*air Density)1/2
  [AHC] -> Room air heat capacity (Cp*volume air*air Density)1/1
  [deltaTextRoof] -> Subsystem3/4(In4)
  RoomNodeNumber1/1 -> Subsystem3/1(In1)
  [T_1] -> Subsystem3/5(In5)
  Subsystem3/4(Out4) -> room deltaT1/1
  Product3/1 -> Subsystem4/7(In7)
  Switch/1 -> Plus/1
  [Floor_U] -> Subsystem5/5(In5)
  Subsystem5/1(Out1) -> Sum2/1
  [RmVol] -> Product2/2
  Product2/1 -> Subsystem5/7(In7)
  [Tin] -> Subsystem5/1(In1)
  [TAbv] -> Subsystem4/3(In3)
  [Cei_U] -> Subsystem5/6(In6)
  Sum1/1 -> Switch/3
  Sum2/1 -> Switch/1
  [Tin] -> Subsystem4/1(In1)
  [AirRHO] -> Product2/3
  Subsystem4/1(Out1) -> Sum1/1
  [TAbv] -> Subsystem5/3(In3)
  [TBel] -> Subsystem5/2(In2)
  [AirRHO] -> Product3/3
  [AHC] -> Product3/1
  [Fl_Area] -> Subsystem4/4(In4)
  Sum5/1 -> [deltaT_Slab]
  [AHC] -> Product2/1
  Subsystem5/2(Out2) -> Sum5/1
  [Fl_Area] -> Subsystem5/4(In4)
  [RmVol] -> Product3/2
  [Floor_U] -> Subsystem4/5(In5)
  [TBel] -> Subsystem4/2(In2)
  [Cei_U] -> Subsystem4/6(In6)
  Constant/1 -> Switch/2
  Integrator26/1 -> Subsystem5/8(In8)
  [deltaT_Slab] -> Integrator26/1
  Twall136/1 -> Integrator26/2
  switc/1 -> Plus/2
  "house has green roof, and the room is on the top floor"/1 -> switc/2, "switches "/2
  Subsystem7/1(Out1) -> switc/1, "switches "/3
  Minus1/1 -> "switches "/1
  "switches "/1 -> switc/3
  Plus/1 -> [deltaT_cond_updown]
  [RmVol] -> Product5/2
  [AHC] -> Product5/1
  [AirRHO] -> Product5/3
  [Occ_Free_Gain] -> deltaT from loss to upstairs1/1
  Product5/1 -> deltaT from loss to upstairs1/2
  deltaT from loss to upstairs1/1 -> Add/8
  [Tin] -> furniture/3(In3)
  Constant2/1 -> furniture/2(In2)
  room deltaT from radiator3/1 -> [deltaT_furniture]
  [AHC] -> Product1/1
  [AirRHO] -> Product1/3
  Constant5/1 -> room deltaT from radiator3/2
  furniture/1(Out1) -> room deltaT from radiator2/1
  room deltaT from radiator2/1 -> room deltaT from radiator3/1
  [Fl_Area] -> furniture/1(In1)
  [RmVol] -> Product1/2
  Product1/1 -> room deltaT from radiator2/2
  [deltaT_furniture] -> Add/3
  Product6/1 -> room deltaT from radiator1/2
  [AirRHO] -> Product6/3
  Subsystem6/1(Out1) -> [Q_rad_win1]
  room deltaT from radiator1/1 -> [deltaT_conv_win]
  [Tout] -> Subsystem6/3(In3)
  Subsystem6/2(Out2) -> room deltaT from radiator1/1
  [Tin] -> Subsystem6/2(In2)
  [RmVol] -> Product6/2
  Constant3/1 -> Subsystem6/1(In1)
  [AHC] -> Product6/1
  [deltaTPartition1] -> Add/9
  [deltaTRoofNodes] -> Subsystem7/2(In2)
  roomNumber/1 -> Subsystem7/1(In1)

== system Final_Model_Building_2_AirflowAdded_BufferMode/Subsystem_Room1/Subsystem11 ==
  In1 : Inport
  In2 : Inport  Port=2
  In3 : Inport  Port=3
  In4 : Inport  Port=4
  Add : Sum
  Add1 : Sum
  Constant : Constant  Value=2
  Constant1 : Constant  Value=2
  Divide : Product  Inputs=*/
  Divide1 : Product  Inputs=*/
  Multiport Switch{,1..3} (4 alike) : MultiPortSwitch  Inputs=14  SaturateOnIntegerOverflow=off  InputSameDT=off
  Out1 : Outport  VectorParamsAs1DForOutWhenUnconnected=off
  Out2 : Outport  Port=2  VectorParamsAs1DForOutWhenUnconnected=off
  wires:
  [T_7] -> Multiport Switch1/8
  [T_1] -> Multiport Switch1/2
  [T_5] -> Multiport Switch/6
  [T_11] -> Multiport Switch1/12
  [T_2] -> Multiport Switch/3
  [T_9] -> Multiport Switch/10
  [T_10] -> Multiport Switch1/11
  [T_10] -> Multiport Switch/11
  [T_3] -> Multiport Switch/4
  [T_12] -> Multiport Switch/13
  [T_3] -> Multiport Switch1/4
  [T_9] -> Multiport Switch1/10
  [T_2] -> Multiport Switch1/3
  [T_11] -> Multiport Switch/12
  [T_12] -> Multiport Switch1/13
  [T_5] -> Multiport Switch1/6
  [T_4] -> Multiport Switch1/5
  [T_4] -> Multiport Switch/5
  [T_1] -> Multiport Switch/2
  [T_8] -> Multiport Switch1/9
  [T_6] -> Multiport Switch1/7
  Multiport Switch/1 -> Add/1
  [T_7] -> Multiport Switch/8
  [T_8] -> Multiport Switch/9
  [T_6] -> Multiport Switch/7
  In2/1 -> Multiport Switch1/1
  Multiport Switch1/1 -> Add/2
  In1/1 -> Multiport Switch/1
  [T_8] -> Multiport Switch2/9
  [T_3] -> Multiport Switch2/4
  [T_2] -> Multiport Switch3/3
  Multiport Switch3/1 -> Add1/2
  [T_10] -> Multiport Switch2/11
  [T_1] -> Multiport Switch2/2
  [T_4] -> Multiport Switch3/5
  [T_9] -> Multiport Switch3/10
  [T_12] -> Multiport Switch3/13
  [T_5] -> Multiport Switch3/6
  [T_6] -> Multiport Switch2/7
  Multiport Switch2/1 -> Add1/1
  [T_4] -> Multiport Switch2/5
  [T_3] -> Multiport Switch3/4
  [T_7] -> Multiport Switch2/8
  [T_11] -> Multiport Switch2/12
  [T_12] -> Multiport Switch2/13
  [T_10] -> Multiport Switch3/11
  [T_6] -> Multiport Switch3/7
  [T_9] -> Multiport Switch2/10
  [T_8] -> Multiport Switch3/9
  [T_11] -> Multiport Switch3/12
  [T_1] -> Multiport Switch3/2
  [T_2] -> Multiport Switch2/3
  [T_5] -> Multiport Switch2/6
  In3/1 -> Multiport Switch2/1
  [T_7] -> Multiport Switch3/8
  In4/1 -> Multiport Switch3/1
  Add/1 -> Divide/1
  Divide/1 -> Out1/1
  Add1/1 -> Divide1/1
  Divide1/1 -> Out2/1
  Constant/1 -> Divide/2
  Constant1/1 -> Divide1/2
  [T_Out] -> Multiport Switch/15
  [T_Out] -> Multiport Switch1/15
  [T_Out] -> Multiport Switch2/15
  [T_Out] -> Multiport Switch3/15
  [Ground] -> Multiport Switch3/14
  [Ground] -> Multiport Switch2/14
  [Ground] -> Multiport Switch1/14
  [Ground] -> Multiport Switch/14

== system Final_Model_Building_2_AirflowAdded_BufferMode/Subsystem_Room1/Subsystem3 ==
  In1 : Inport
  In2 : Inport  Port=2
  In3 : Inport  Port=3
  In4 : Inport  Port=4
  In5 : Inport  Port=5
  Multiport Switch{,1..4} (5 alike) : MultiPortSwitch  Inputs=12  SaturateOnIntegerOverflow=off  InputSameDT=off
  Out1 : Outport  VectorParamsAs1DForOutWhenUnconnected=off
  Out2 : Outport  Port=2  VectorParamsAs1DForOutWhenUnconnected=off
  Out3 : Outport  Port=3  VectorParamsAs1DForOutWhenUnconnected=off
  Out4 : Outport  Port=4  VectorParamsAs1DForOutWhenUnconnected=off
  Out5 : Outport  Port=5  VectorParamsAs1DForOutWhenUnconnected=off
  wires:
  [T_7] -> Multiport Switch1/8
  In5/1 -> Multiport Switch4/1
  [T_1] -> Multiport Switch1/2
  [T_5] -> Multiport Switch/6
  [T_3] -> Multiport Switch2/4
  [T_9] -> Multiport Switch2/10
  [T_10] -> Multiport Switch3/11
  [T_11] -> Multiport Switch1/12
  [T_2] -> Multiport Switch/3
  [T_9] -> Multiport Switch/10
  [T_10] -> Multiport Switch1/11
  [T_10] -> Multiport Switch/11
  [T_9] -> Multiport Switch4/10
  [T_11] -> Multiport Switch2/12
  [T_3] -> Multiport Switch/4
  [T_12] -> Multiport Switch/13
  [T_7] -> Multiport Switch2/8
  [T_4] -> Multiport Switch3/5
  [T_10] -> Multiport Switch2/11
  [T_2] -> Multiport Switch4/3
  [T_3] -> Multiport Switch1/4
  [T_9] -> Multiport Switch1/10
  [T_2] -> Multiport Switch1/3
  [T_6] -> Multiport Switch3/7
  [T_11] -> Multiport Switch/12
  [T_8] -> Multiport Switch2/9
  [T_12] -> Multiport Switch1/13
  [T_7] -> Multiport Switch3/8
  [T_5] -> Multiport Switch1/6
  [T_6] -> Multiport Switch2/7
  [T_4] -> Multiport Switch1/5
  [T_4] -> Multiport Switch/5
  [T_1] -> Multiport Switch/2
  [T_8] -> Multiport Switch1/9
  [T_10] -> Multiport Switch4/11
  [T_6] -> Multiport Switch1/7
  In4/1 -> Multiport Switch3/1
  Multiport Switch/1 -> Out1/1
  [T_5] -> Multiport Switch2/6
  [T_7] -> Multiport Switch/8
  [T_8] -> Multiport Switch3/9
  Multiport Switch2/1 -> Out3/1
  [T_4] -> Multiport Switch2/5
  [T_8] -> Multiport Switch/9
  [T_12] -> Multiport Switch3/13
  [T_6] -> Multiport Switch/7
  [T_8] -> Multiport Switch4/9
  [T_2] -> Multiport Switch3/3
  [T_11] -> Multiport Switch3/12
  [T_1] -> Multiport Switch3/2
  [T_11] -> Multiport Switch4/12
  [T_2] -> Multiport Switch2/3
  [T_3] -> Multiport Switch3/4
  [T_12] -> Multiport Switch2/13
  In2/1 -> Multiport Switch1/1
  [T_9] -> Multiport Switch3/10
  [T_5] -> Multiport Switch3/6
  [T_1] -> Multiport Switch4/2
  [T_3] -> Multiport Switch4/4
  [T_12] -> Multiport Switch4/13
  [T_6] -> Multiport Switch4/7
  [T_4] -> Multiport Switch4/5
  [T_7] -> Multiport Switch4/8
  [T_5] -> Multiport Switch4/6
  [T_1] -> Multiport Switch2/2
  Multiport Switch1/1 -> Out2/1
  Multiport Switch3/1 -> Out4/1
  In3/1 -> Multiport Switch2/1
  Multiport Switch4/1 -> Out5/1
  In1/1 -> Multiport Switch/1
